simulink model "testTurningMachine"  (R2023a)
settings: Solver=VariableStepAuto  StartTime=0.0  StopTime=10.0  RelTol=1e-3
libraries: NSA_DEVS_SINKS x8, NSA_DEVS_LOGISTICS x3, ProductionLineLib_CM x1
settings Model: Creator=peter  LastModifiedBy=peter

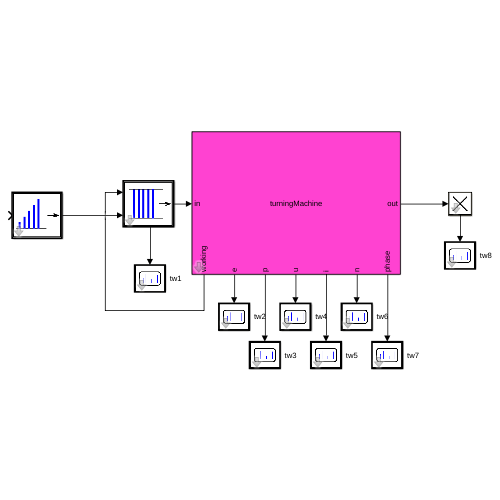
[thumbnail: Simulink's stored preview of the top-level diagram]
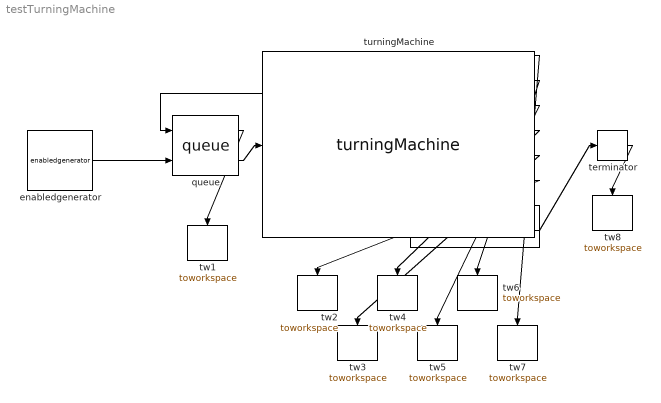
== system testTurningMachine ==
  enabledgenerator : NSA_DEVS_LOGISTICS/enabledgenerator  tG=3000  n0=0  nG=4  tau=[0,1]  debug=0
      settings: SourceProductName=NSA_DEVS
  queue : NSA_DEVS_LOGISTICS/queue  tD=[0,5]  tau=[0,5]  debug=0
      settings: SourceProductName=NSA_DEVS
  terminator : NSA_DEVS_LOGISTICS/terminator  tau=[0,1]  debug=0
      settings: SourceProductName=NSA_DEVS
  turningMachine : ProductionLineLib_CM/turningMachine  turning_time=20*60  ap_ug=0.5  ap_og=1.5  P_ap=0.6  f_ug=0.1  f_og=0.5  P_f=0.4  vc_ug=150  vc_og=350  P_vc=0.5  ap=0  f=0  vc=0  tauInt=[0,100]  tauCont=[0,100]  tau=[0,1]  debug=0
      settings: LibrarySourceBlock=ProductionLineLib_CM/turning
  tw1 : NSA_DEVS_SINKS/toworkspace  varname="\"nq\""  t0=0  format="\"vector\""  tau=[0,1]  debug=0
      settings: SourceProductName=NSA_DEVS
  tw2 : NSA_DEVS_SINKS/toworkspace  varname="\"E\""  t0=0  format="\"vector\""  tau=[0,1]  debug=0
      settings: SourceProductName=NSA_DEVS
  tw3 : NSA_DEVS_SINKS/toworkspace  varname="\"P\""  t0=0  format="\"vector\""  tau=[0,1]  debug=0
      settings: SourceProductName=NSA_DEVS
  tw4 : NSA_DEVS_SINKS/toworkspace  varname="\"u\""  t0=0  format="\"vector\""  tau=[0,1]  debug=0
      settings: SourceProductName=NSA_DEVS
  tw5 : NSA_DEVS_SINKS/toworkspace  varname="\"i\""  t0=0  format="\"vector\""  tau=[0,1]  debug=0
      settings: SourceProductName=NSA_DEVS
  tw6 : NSA_DEVS_SINKS/toworkspace  varname="\"n\""  t0=0  format="\"vector\""  tau=[0,1]  debug=0
      settings: SourceProductName=NSA_DEVS
  tw7 : NSA_DEVS_SINKS/toworkspace  varname="\"phase\""  t0=0  format="\"vector\""  tau=[0,1]  debug=0
      settings: SourceProductName=NSA_DEVS
  tw8 : NSA_DEVS_SINKS/toworkspace  varname="\"nout\""  t0=0  format="\"vector\""  tau=[0,1]  debug=0
      settings: SourceProductName=NSA_DEVS
  wires:
  enabledgenerator/1 -> queue/1
  turningMachine/1 -> terminator/1
  turningMachine/2 -> queue/2
  queue/1 -> turningMachine/1
  queue/2 -> tw1/1
  terminator/1 -> tw8/1
  turningMachine/3 -> tw2/1
  turningMachine/4 -> tw3/1
  turningMachine/5 -> tw4/1
  turningMachine/6 -> tw5/1
  turningMachine/7 -> tw6/1
  turningMachine/8 -> tw7/1
